simulink library "DistanceSensor"  (R2018b)
settings: Solver=VariableStepAuto  StartTime=0.0  StopTime=10.0  RelTol=1e-3
settings Model: Creator=nico  LastModifiedBy=nico

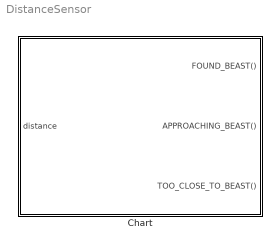
== system DistanceSensor ==
  Chart : Stateflow chart  TreatAsAtomicUnit=on

== stateflow chart DistanceSensor/Chart ==
  state TooClose
    entry:
    send(TOO_CLOSE_TO_BEAST)
  state Approached
    entry:
    send(FOUND_BEAST)
  state Approaching
    entry:
    send(APPROACHING_BEAST)
  state Start
  (default) -> Start
  Approached -> TooClose [order 1] : [distance < 10]
  Approaching -> Approached : [distance <= 12]
  Start -> Approaching : [distance < 255]
  Approached -> Approaching [order 2] : [distance > 12]
  TooClose -> Approached : [distance >= 10]
  data: distance input
  events: FOUND_BEAST output FUNCTION_CALL_EVENT; APPROACHING_BEAST output FUNCTION_CALL_EVENT; TOO_CLOSE_TO_BEAST output FUNCTION_CALL_EVENT
